simulink model "nms_3Dmodel_inv_wAnkleCPG"  (R2016b)
settings: Solver=ode3  StartTime=0.0  StopTime=tend  FixedStep=ts  RelTol=1e-3  EnableMultiTasking=on
InitFcn:
  | runScripts_inv;
values from neighbouring files (symbols this model uses):
  c = 0.05    [IID_nms_MechInit.m]    (also in nms_MechInit.m)
  c_jointstop = 0.3 / (pi/180)    (= 17.1887338539)    [IID_nms_MechInit.m]    (also in nms_MechInit.m)
  CPG_On = 1    [setCPGPar.m]    (also in setCPGPar_inv.m)
  CtrlPar_FP = [alpha0 alpha_cd alpha_cv]    [setCtrlPar.m]
  CtrlPar_FP_R = [R_hipR0 R_hipR_cd R_hipR_cv]    [setCtrlPar.m]
  CtrlPar_LL = l_clr    [setCtrlPar.m]
  CtrlPar_St = [StPreStim St_M1 St_M2 St_M3 St_M4 St_M5 St_M11]    [setCtrlPar.m]
  CtrlPar_St_R = [R_StPreStim R_St_M1 R_St_M3 R_St_M4]    [setCtrlPar.m]
  CtrlPar_Sw = [SwPreStim SwPhasePari SwPhaseParii SwCtrlPar_H SwCtrlPar_A      SwCtrlPar_Ki SwCtrlPar_Kii SwCtrlPar_Kiii SwCtrlPar_StP]    [setCtrlPar.m]
  CtrlPar_Sw_R = [R_SwPreStim R_Sw_M6]    [setCtrlPar.m]
  CtrlPar_theta0 = parBlCtrl(1)      *1*pi/180    [setCtrlPar.m]
  CtrlPar_Tr = [Tr_St_sup Tr_Sw]    [setCtrlPar.m]
  CtrlPar_Tr_R = [R_Tr_St_sup R_Tr_Sw]    [setCtrlPar.m]
  eref = 0.04    [IID_nms_MechInit.m]    (also in nms_MechInit.m)
  FmaxBFSH = 350    [nms_MechInit.m]
  FmaxGAS = 1500    [IID_nms_MechInit.m]    (also in nms_MechInit.m)
  FmaxGLU = 1500    [IID_nms_MechInit.m]    (also in nms_MechInit.m)
  FmaxHAB = 3000    [nms_MechInit.m]
  FmaxHAD = 4500    [nms_MechInit.m]
  FmaxHAM = 3000    [IID_nms_MechInit.m]    (also in nms_MechInit.m)
  FmaxHFL = 2000    [IID_nms_MechInit.m]    (also in nms_MechInit.m)
  FmaxRF = 1200    [nms_MechInit.m]
  FmaxSOL = 4000    [IID_nms_MechInit.m]    (also in nms_MechInit.m)
  FmaxTA = 800    [IID_nms_MechInit.m]    (also in nms_MechInit.m)
  FmaxVAS = 6000    [IID_nms_MechInit.m]    (also in nms_MechInit.m)
  init_a_tgt = 70*pi/180    (= 1.2217304764)    [setInitPar.m]
  init_a_tgtR = 90*pi/180    (= 1.57079632679)    [setInitPar.m]
  K = 5    [IID_nms_MechInit.m]    (also in nms_MechInit.m)
  leg_l = [D12_T D12_S]    [nms_MechInit.m]
  LongDelay = 0.020    (= 0.02)    [IID_setCtrlPar.m]    (also in nms_MechInit.m = 0.01)
  LongLoopDelay = 0.030    (= 0.03)    [nms_MechInit.m]
  loptBFSH = 0.12    [nms_MechInit.m]
  loptGAS = 0.05    [IID_nms_MechInit.m]    (also in nms_MechInit.m)
  loptGLU = 0.11    [IID_nms_MechInit.m]    (also in nms_MechInit.m)
  loptHAB = 0.09    [nms_MechInit.m]
  loptHAD = 0.10    (= 0.1)    [nms_MechInit.m]
  loptHAM = 0.10    (= 0.1)    [IID_nms_MechInit.m]    (also in nms_MechInit.m)
  loptHFL = 0.11    [IID_nms_MechInit.m]    (also in nms_MechInit.m)
  loptRF = 0.08    [nms_MechInit.m]
  loptSOL = 0.04    [IID_nms_MechInit.m]    (also in nms_MechInit.m)
  loptTA = 0.06    [IID_nms_MechInit.m]    (also in nms_MechInit.m)
  loptVAS = 0.08    [IID_nms_MechInit.m]    (also in nms_MechInit.m)
  lslackBFSH = 0.10    (= 0.1)    [nms_MechInit.m]
  lslackGAS = 0.40    (= 0.4)    [IID_nms_MechInit.m]    (also in nms_MechInit.m)
  lslackGLU = 0.13    [IID_nms_MechInit.m]    (also in nms_MechInit.m)
  lslackHAB = 0.07    [nms_MechInit.m]
  lslackHAD = 0.18    [nms_MechInit.m]
  lslackHAM = 0.31    [IID_nms_MechInit.m]    (also in nms_MechInit.m)
  lslackHFL = 0.10    (= 0.1)    [IID_nms_MechInit.m]    (also in nms_MechInit.m)
  lslackRF = 0.35    [nms_MechInit.m]
  lslackSOL = 0.26    [IID_nms_MechInit.m]    (also in nms_MechInit.m)
  lslackTA = 0.24    [IID_nms_MechInit.m]    (also in nms_MechInit.m)
  lslackVAS = 0.23    [IID_nms_MechInit.m]    (also in nms_MechInit.m)
  massBFSH = 2    [nms_MechInit.m]
  massGAS = 0.45    [IID_nms_MechInit.m]    (also in nms_MechInit.m)
  massGLU = 1.4    [IID_nms_MechInit.m]    (also in nms_MechInit.m)
  massHAB = 1.145    [nms_MechInit.m]
  massHAD = 1.91    [nms_MechInit.m]
  massHAM = 1.82    [IID_nms_MechInit.m]    (also in nms_MechInit.m)
  massHFL = 1.87    [IID_nms_MechInit.m]    (also in nms_MechInit.m)
  massRF = 1    [nms_MechInit.m]
  massSOL = 1.36    [IID_nms_MechInit.m]    (also in nms_MechInit.m)
  massTA = 0.29    [IID_nms_MechInit.m]    (also in nms_MechInit.m)
  massVAS = 2.91    [IID_nms_MechInit.m]    (also in nms_MechInit.m)
  MidDelay = 0.010    (= 0.01)    [IID_setCtrlPar.m]    (also in nms_MechInit.m = 0.005)
  N = 1.5    [IID_nms_MechInit.m]    (also in cmaes_parfor.m = size(x,1); nms_MechInit.m)
  phi12_LowLimit = 70*pi/180    (= 1.2217304764)    [IID_nms_MechInit.m]    (also in nms_MechInit.m)
  phi12_UpLimit = 130*pi/180    (= 2.26892802759)    [IID_nms_MechInit.m]    (also in nms_MechInit.m)
  phi23_UpLimit = 175*pi/180    (= 3.05432619099)    [IID_nms_MechInit.m]    (also in nms_MechInit.m)
  phi34_UpLimit = 230*pi/180    (= 4.01425727959)    [IID_nms_MechInit.m]    (also in nms_MechInit.m)
  phi34R_LowLimit = -15*pi/180    (= -0.261799387799)    [nms_MechInit.m]
  phi34R_UpLimit = 50*pi/180    (= 0.872664625997)    [nms_MechInit.m]
  phimaxGASa = 110*pi/180    (= 1.91986217719)    [IID_nms_MechInit.m]    (also in nms_MechInit.m = 1.74532925199)
  phimaxGASk = 140*pi/180    (= 2.44346095279)    [IID_nms_MechInit.m]    (also in nms_MechInit.m)
  phimaxRFk = 165*pi/180    (= 2.87979326579)    [nms_MechInit.m]
  phimaxSOL = 110*pi/180    (= 1.91986217719)    [IID_nms_MechInit.m]    (also in nms_MechInit.m = 1.74532925199)
  phimaxTA = 80*pi/180    (= 1.3962634016)    [IID_nms_MechInit.m]    (also in nms_MechInit.m)
  phimaxVAS = 165*pi/180    (= 2.87979326579)    [IID_nms_MechInit.m]    (also in nms_MechInit.m)
  phirefBFSH = 160*pi/180    (= 2.79252680319)    [nms_MechInit.m]
  phirefGASa = 80*pi/180    (= 1.3962634016)    [IID_nms_MechInit.m]    (also in nms_MechInit.m)
  phirefGASk = 165*pi/180    (= 2.87979326579)    [IID_nms_MechInit.m]    (also in nms_MechInit.m)
  phirefGLU = 150*pi/180    (= 2.61799387799)    [IID_nms_MechInit.m]    (also in nms_MechInit.m = 2.09439510239)
  phirefHAB = 10*pi/180    (= 0.174532925199)    [nms_MechInit.m]
  phirefHAD = 15*pi/180    (= 0.261799387799)    [nms_MechInit.m]
  phirefHAMh = 155*pi/180    (= 2.70526034059)    [IID_nms_MechInit.m]    (also in nms_MechInit.m = 2.61799387799)
  phirefHAMk = 180*pi/180    (= 3.14159265359)    [IID_nms_MechInit.m]    (also in nms_MechInit.m)
  phirefHFL = 180*pi/180    (= 3.14159265359)    [IID_nms_MechInit.m]    (also in nms_MechInit.m = 2.79252680319)
  phirefRFh = 170*pi/180    (= 2.96705972839)    [nms_MechInit.m]
  phirefRFk = 125*pi/180    (= 2.18166156499)    [nms_MechInit.m]
  phirefSOL = 80*pi/180    (= 1.3962634016)    [IID_nms_MechInit.m]    (also in nms_MechInit.m = 1.57079632679)
  phirefTA = 110*pi/180    (= 1.91986217719)    [IID_nms_MechInit.m]    (also in nms_MechInit.m)
  phirefVAS = 125*pi/180    (= 2.18166156499)    [IID_nms_MechInit.m]    (also in nms_MechInit.m = 2.09439510239)
  phiScaleGASa = acos(rGASamin/rGASamax)/(phiminGASa-phimaxGASa)    [nms_MechInit.m]
  phiScaleGASk = acos(rGASkmin/rGASkmax)/(phiminGASk-phimaxGASk)    [nms_MechInit.m]
  phiScaleRFk = acos(rRFkmin/rRFkmax)/(phiminRFk-phimaxRFk)    [nms_MechInit.m]
  phiScaleSOL = acos(rSOLmin/rSOLmax)/(phiminSOL-phimaxSOL)    [nms_MechInit.m]
  phiScaleTA = acos(rTAmin/rTAmax)/(phiminTA-phimaxTA)    [nms_MechInit.m]
  phiScaleVAS = acos(rVASmin/rVASmax)/(phiminVAS-phimaxVAS)    [nms_MechInit.m]
  rBFSH = 0.04    [nms_MechInit.m]
  rGASamax = 0.06    [nms_MechInit.m]
  rGASkmax = 0.05    [nms_MechInit.m]
  rGLU = 0.10    (= 0.1)    [IID_nms_MechInit.m]    (also in nms_MechInit.m = 0.08)
  rHAB = 0.06    [nms_MechInit.m]
  rHAD = 0.03    [nms_MechInit.m]
  rHAMh = 0.08    [IID_nms_MechInit.m]    (also in nms_MechInit.m)
  rHAMk = 0.05    [IID_nms_MechInit.m]    (also in nms_MechInit.m)
  rHFL = 0.10    (= 0.1)    [IID_nms_MechInit.m]    (also in nms_MechInit.m = 0.08)
  rhoBFSH = 0.7    [nms_MechInit.m]
  rhoGASa = 0.7    [IID_nms_MechInit.m]    (also in nms_MechInit.m)
  rhoGASk = 0.7    [IID_nms_MechInit.m]    (also in nms_MechInit.m)
  rhoGLU = 0.5    [IID_nms_MechInit.m]    (also in nms_MechInit.m)
  rhoHAB = 0.7    [nms_MechInit.m]
  rhoHAD = 1    [nms_MechInit.m]
  rhoHAMh = 0.7    [IID_nms_MechInit.m]    (also in nms_MechInit.m = 0.5)
  rhoHAMk = 0.7    [IID_nms_MechInit.m]    (also in nms_MechInit.m = 0.5)
  rhoHFL = 0.5    [IID_nms_MechInit.m]    (also in nms_MechInit.m)
  rhoRFh = 0.3    [nms_MechInit.m]
  rhoRFk = 0.5    [nms_MechInit.m]
  rhoSOL = 0.5    [IID_nms_MechInit.m]    (also in nms_MechInit.m)
  rhoTA = 0.7    [IID_nms_MechInit.m]    (also in nms_MechInit.m)
  ... (+55 more)
libraries: simulink_extras x30, nmc x30, simulink x22, NMCCPG_Library x13, powerlib_meascontrol x5
(part 4 of 12)

== system nms_3Dmodel_inv_wAnkleCPG/NMC Model/Muscle Actuation Layer/L GLU ==
  note: Excitation Contraction Coupling
  note: GLU Muscle-Tendon Dynamics
  STIM : Inport
  lmtc [m] : Inport  Port=2
  1 : Product  Inputs=**  SaturateOnIntegerOverflow=on  InputSameDT=on  OutDataTypeStr=Inherit: Same as first input
  1/lslack : Gain  Gain=1/lslackGLU  SaturateOnIntegerOverflow=on  OutDataTypeStr=Inherit: Same as input  ParamDataTypeStr=Inherit: Same as input
  2 : Product  Inputs=***  SaturateOnIntegerOverflow=on  InputSameDT=on  OutDataTypeStr=Inherit: Same as first input
  BE force-length relation : Subsystem
  CE force-length relation : Subsystem
  CE inverse force-velocity relation : Subsystem
  Constant : Constant  Value=lslackGLU
  ECC TransferFcn : simulink_extras/Additional Linear/Transfer Fcn (with initial outputs)  N=[1]  D="[tau  1]"  Y0=preA  U0=0
      settings: AttributesFormatString=pre-activation: %<Y0>
  Fmax : Gain  Gain=FmaxGLU  SaturateOnIntegerOverflow=on  OutDataTypeStr=Inherit: Same as input  ParamDataTypeStr=Inherit: Same as input
  Fmax1 : Gain  Gain=FmaxGLU  SaturateOnIntegerOverflow=on  OutDataTypeStr=Inherit: Same as input  ParamDataTypeStr=Inherit: Same as input
  Fv = Fse / (A*Fce) : Product  Inputs=*/  SaturateOnIntegerOverflow=on  InputSameDT=on  OutDataTypeStr=Inherit: Same as first input
  Integrator : Integrator  InitialConditionSource=external  LowerSaturationLimit=0.05  ZeroCross=off
  PE force-length relation : Subsystem
  SE force-length relation : Subsystem
  Sum : Sum  Inputs=|+-  SaturateOnIntegerOverflow=on  InputSameDT=on  OutDataTypeStr=Inherit: Same as first input
  Sum2 : Sum  Inputs=|-+  SaturateOnIntegerOverflow=on  InputSameDT=on  OutDataTypeStr=Inherit: Same as first input
  Sum3 : Sum  SaturateOnIntegerOverflow=on  InputSameDT=on  OutDataTypeStr=Inherit: Same as first input
  Sum4 : Sum  SaturateOnIntegerOverflow=on  InputSameDT=on  OutDataTypeStr=Inherit: Same as first input
  lce/lopt : Gain  Gain=1/loptGLU  SaturateOnIntegerOverflow=on  OutDataTypeStr=Inherit: Same as input  ParamDataTypeStr=Inherit: Same as input
  vmax*lopt : Gain  Gain=vmaxGLU*loptGLU  SaturateOnIntegerOverflow=on  OutDataTypeStr=Inherit: Same as input  ParamDataTypeStr=Inherit: Same as input
  Fmtc : Outport  InitialOutput=0
  Lce : Outport  Port=2  InitialOutput=0
  Vce : Outport  Port=3  InitialOutput=0
  A : Outport  Port=4  InitialOutput=0
  Fac : Outport  Port=5  InitialOutput=0
  wires:
  Fmax1/1 -> Fac/1
  2/1 -> Fmax1/1
  ECC TransferFcn/1 -> 1/2, A/1, 2/2  "A"
  CE force-length relation/1(fce [Fmax]) -> 1/1, 2/1  "fl"
  Fv = Fse / (A*Fce)/1 -> CE inverse force-velocity relation/1(Fv[Fmax]), 2/3  "fv"
  STIM/1 -> ECC TransferFcn/1
  CE inverse force-velocity relation/1(v[vmax]) -> vmax*lopt/1
  Sum3/1 -> Fv = Fse / (A*Fce)/2
  BE force-length relation/1(fbe [Fmax]) -> Sum4/2
  1/1 -> Sum3/2
  PE force-length relation/1(fpe [Fmax]) -> Sum3/1
  Sum4/1 -> Fv = Fse / (A*Fce)/1
  Constant/1 -> Sum2/1
  Sum2/1 -> Integrator/2
  SE force-length relation/1(fse [Fmax]) -> Sum4/1, Fmax/1
  1/lslack/1 -> SE force-length relation/1(lse [lslack])
  Fmax/1 -> Fmtc/1  "Fmtc"
  lmtc [m]/1 -> Sum/1, Sum2/2  "lmtc"
  vmax*lopt/1 -> Vce/1, Integrator/1  "vce"
  lce/lopt/1 -> PE force-length relation/1(lce [lopt]), BE force-length relation/1(lce [lopt]), CE force-length relation/1(lce [lopt])
  Sum/1 -> 1/lslack/1  "lse"
  Integrator/1 -> Lce/1, lce/lopt/1, Sum/2  "lce"

== system nms_3Dmodel_inv_wAnkleCPG/NMC Model/Muscle Actuation Layer/L GLU Link ==
  note: GLUTEUS Attachment
  phi34 [rad] : Inport
  Constant : Constant  Value=lslackGLU+loptGLU
  Constant1 : Constant  Value=rGLU
  Constant2 : Constant  Value=phirefGLU
  Gain2 : Gain  Gain=rhoGLU
  Product : Product  RndMeth=Zero
  Sum2 : Sum  Inputs=|+-
  Sum5 : Sum  Inputs=|+-
  lmtu [m] : Outport
  lever [m] : Outport  Port=2
  wires:
  Gain2/1 -> Sum5/2
  Constant1/1 -> lever [m]/1, Product/2
  Sum2/1 -> Product/1
  Constant2/1 -> Sum2/2
  phi34 [rad]/1 -> Sum2/1
  Product/1 -> Gain2/1
  Sum5/1 -> lmtu [m]/1
  Constant/1 -> Sum5/1

== system nms_3Dmodel_inv_wAnkleCPG/NMC Model/Muscle Actuation Layer/L HAB ==
  note: HAB Muscle-Tendon Dynamics
  note: Excitation Contraction Coupling
  STIM : Inport
  lmtc [m] : Inport  Port=2
  1 : Product  Inputs=**  SaturateOnIntegerOverflow=on  InputSameDT=on  OutDataTypeStr=Inherit: Same as first input
  1/lslack : Gain  Gain=1/lslackHAB  SaturateOnIntegerOverflow=on  OutDataTypeStr=Inherit: Same as input  ParamDataTypeStr=Inherit: Same as input
  2 : Product  Inputs=***  SaturateOnIntegerOverflow=on  InputSameDT=on  OutDataTypeStr=Inherit: Same as first input
  BE force-length relation : Subsystem
  CE force-length relation : Subsystem
  CE inverse force-velocity relation : Subsystem
  Constant : Constant  Value=lslackHAB
  ECC TransferFcn : simulink_extras/Additional Linear/Transfer Fcn (with initial outputs)  N=[1]  D="[tau  1]"  Y0=preA  U0=0
      settings: AttributesFormatString=pre-activation: %<Y0>
  Fmax : Gain  Gain=FmaxHAB  SaturateOnIntegerOverflow=on  OutDataTypeStr=Inherit: Same as input  ParamDataTypeStr=Inherit: Same as input
  Fmax1 : Gain  Gain=FmaxHAB  SaturateOnIntegerOverflow=on  OutDataTypeStr=Inherit: Same as input  ParamDataTypeStr=Inherit: Same as input
  Fv = Fse / (A*Fce) : Product  Inputs=*/  SaturateOnIntegerOverflow=on  InputSameDT=on  OutDataTypeStr=Inherit: Same as first input
  Integrator : Integrator  InitialConditionSource=external  LowerSaturationLimit=0.05  ZeroCross=off
  PE force-length relation : Subsystem
  SE force-length relation : Subsystem
  Sum : Sum  Inputs=|+-  SaturateOnIntegerOverflow=on  InputSameDT=on  OutDataTypeStr=Inherit: Same as first input
  Sum2 : Sum  Inputs=|-+  SaturateOnIntegerOverflow=on  InputSameDT=on  OutDataTypeStr=Inherit: Same as first input
  Sum3 : Sum  SaturateOnIntegerOverflow=on  InputSameDT=on  OutDataTypeStr=Inherit: Same as first input
  Sum4 : Sum  SaturateOnIntegerOverflow=on  InputSameDT=on  OutDataTypeStr=Inherit: Same as first input
  lce/lopt : Gain  Gain=1/loptHAB  SaturateOnIntegerOverflow=on  OutDataTypeStr=Inherit: Same as input  ParamDataTypeStr=Inherit: Same as input
  vmax*lopt : Gain  Gain=vmaxHAB*loptHAB  SaturateOnIntegerOverflow=on  OutDataTypeStr=Inherit: Same as input  ParamDataTypeStr=Inherit: Same as input
  Fmtc : Outport  InitialOutput=0
  Lce : Outport  Port=2  InitialOutput=0
  Vce : Outport  Port=3  InitialOutput=0
  A : Outport  Port=4  InitialOutput=0
  Fac : Outport  Port=5  InitialOutput=0
  wires:
  Integrator/1 -> Sum/2, lce/lopt/1, Lce/1  "lce"
  Sum/1 -> 1/lslack/1  "lse"
  lce/lopt/1 -> CE force-length relation/1(lce [lopt]), BE force-length relation/1(lce [lopt]), PE force-length relation/1(lce [lopt])
  vmax*lopt/1 -> Integrator/1, Vce/1  "vce"
  lmtc [m]/1 -> Sum2/2, Sum/1  "lmtc"
  Fmax/1 -> Fmtc/1  "Fmtc"
  1/lslack/1 -> SE force-length relation/1(lse [lslack])
  SE force-length relation/1(fse [Fmax]) -> Fmax/1, Sum4/1
  Sum2/1 -> Integrator/2
  Constant/1 -> Sum2/1
  Sum4/1 -> Fv = Fse / (A*Fce)/1
  PE force-length relation/1(fpe [Fmax]) -> Sum3/1
  1/1 -> Sum3/2
  BE force-length relation/1(fbe [Fmax]) -> Sum4/2
  Sum3/1 -> Fv = Fse / (A*Fce)/2
  CE inverse force-velocity relation/1(v[vmax]) -> vmax*lopt/1
  STIM/1 -> ECC TransferFcn/1
  Fv = Fse / (A*Fce)/1 -> 2/3, CE inverse force-velocity relation/1(Fv[Fmax])  "fv"
  CE force-length relation/1(fce [Fmax]) -> 2/1, 1/1  "fl"
  ECC TransferFcn/1 -> 2/2, A/1, 1/2  "A"
  2/1 -> Fmax1/1
  Fmax1/1 -> Fac/1

== system nms_3Dmodel_inv_wAnkleCPG/NMC Model/Muscle Actuation Layer/L HAB Link ==
  note: HAB Attachment
  phi34R [rad] : Inport
  Constant : Constant  Value=lslackHAB+loptHAB
  Constant1 : Constant  Value=rHAB
  Constant2 : Constant  Value=phirefHAB
  Gain2 : Gain  Gain=rhoHAB
  Product : Product  RndMeth=Zero
  Sum2 : Sum  Inputs=|+-
  Sum5 : Sum  Inputs=|+-
  lmtu [m] : Outport
  lever [m] : Outport  Port=2
  wires:
  Gain2/1 -> Sum5/2
  Constant1/1 -> lever [m]/1, Product/2
  Sum2/1 -> Product/1
  Constant2/1 -> Sum2/2
  phi34R [rad]/1 -> Sum2/1
  Product/1 -> Gain2/1
  Sum5/1 -> lmtu [m]/1
  Constant/1 -> Sum5/1

== system nms_3Dmodel_inv_wAnkleCPG/NMC Model/Muscle Actuation Layer/L HAD ==
  note: HAD Muscle-Tendon Dynamics
  note: Excitation Contraction Coupling
  STIM : Inport
  lmtc [m] : Inport  Port=2
  1 : Product  Inputs=**  SaturateOnIntegerOverflow=on  InputSameDT=on  OutDataTypeStr=Inherit: Same as first input
  1/lslack : Gain  Gain=1/lslackHAD  SaturateOnIntegerOverflow=on  OutDataTypeStr=Inherit: Same as input  ParamDataTypeStr=Inherit: Same as input
  2 : Product  Inputs=***  SaturateOnIntegerOverflow=on  InputSameDT=on  OutDataTypeStr=Inherit: Same as first input
  BE force-length relation : Subsystem
  CE force-length relation : Subsystem
  CE inverse force-velocity relation : Subsystem
  Constant : Constant  Value=lslackHAD
  ECC TransferFcn : simulink_extras/Additional Linear/Transfer Fcn (with initial outputs)  N=[1]  D="[tau  1]"  Y0=preA  U0=0
      settings: AttributesFormatString=pre-activation: %<Y0>
  Fmax : Gain  Gain=FmaxHAD  SaturateOnIntegerOverflow=on  OutDataTypeStr=Inherit: Same as input  ParamDataTypeStr=Inherit: Same as input
  Fmax1 : Gain  Gain=FmaxHAD  SaturateOnIntegerOverflow=on  OutDataTypeStr=Inherit: Same as input  ParamDataTypeStr=Inherit: Same as input
  Fv = Fse / (A*Fce) : Product  Inputs=*/  SaturateOnIntegerOverflow=on  InputSameDT=on  OutDataTypeStr=Inherit: Same as first input
  Integrator : Integrator  InitialConditionSource=external  LowerSaturationLimit=0.05  ZeroCross=off
  PE force-length relation : Subsystem
  SE force-length relation : Subsystem
  Sum : Sum  Inputs=|+-  SaturateOnIntegerOverflow=on  InputSameDT=on  OutDataTypeStr=Inherit: Same as first input
  Sum2 : Sum  Inputs=|-+  SaturateOnIntegerOverflow=on  InputSameDT=on  OutDataTypeStr=Inherit: Same as first input
  Sum3 : Sum  SaturateOnIntegerOverflow=on  InputSameDT=on  OutDataTypeStr=Inherit: Same as first input
  Sum4 : Sum  SaturateOnIntegerOverflow=on  InputSameDT=on  OutDataTypeStr=Inherit: Same as first input
  lce/lopt : Gain  Gain=1/loptHAD  SaturateOnIntegerOverflow=on  OutDataTypeStr=Inherit: Same as input  ParamDataTypeStr=Inherit: Same as input
  vmax*lopt : Gain  Gain=vmaxHAD*loptHAD  SaturateOnIntegerOverflow=on  OutDataTypeStr=Inherit: Same as input  ParamDataTypeStr=Inherit: Same as input
  Fmtc : Outport  InitialOutput=0
  Lce : Outport  Port=2  InitialOutput=0
  Vce : Outport  Port=3  InitialOutput=0
  A : Outport  Port=4  InitialOutput=0
  Fac : Outport  Port=5  InitialOutput=0
  wires:
  Integrator/1 -> Sum/2, lce/lopt/1, Lce/1  "lce"
  Sum/1 -> 1/lslack/1  "lse"
  lce/lopt/1 -> CE force-length relation/1(lce [lopt]), BE force-length relation/1(lce [lopt]), PE force-length relation/1(lce [lopt])
  vmax*lopt/1 -> Integrator/1, Vce/1  "vce"
  lmtc [m]/1 -> Sum2/2, Sum/1  "lmtc"
  Fmax/1 -> Fmtc/1  "Fmtc"
  1/lslack/1 -> SE force-length relation/1(lse [lslack])
  SE force-length relation/1(fse [Fmax]) -> Fmax/1, Sum4/1
  Sum2/1 -> Integrator/2
  Constant/1 -> Sum2/1
  CE force-length relation/1(fce [Fmax]) -> 2/1, 1/1
  Sum4/1 -> Fv = Fse / (A*Fce)/1
  PE force-length relation/1(fpe [Fmax]) -> Sum3/1
  1/1 -> Sum3/2
  BE force-length relation/1(fbe [Fmax]) -> Sum4/2
  Sum3/1 -> Fv = Fse / (A*Fce)/2
  CE inverse force-velocity relation/1(v[vmax]) -> vmax*lopt/1
  STIM/1 -> ECC TransferFcn/1
  Fv = Fse / (A*Fce)/1 -> 2/3, CE inverse force-velocity relation/1(Fv[Fmax])  "fv"
  ECC TransferFcn/1 -> 2/2, A/1, 1/2  "A"
  2/1 -> Fmax1/1
  Fmax1/1 -> Fac/1

== system nms_3Dmodel_inv_wAnkleCPG/NMC Model/Muscle Actuation Layer/L HAD Link ==
  note: HAD Attachment
  phi34R [rad] : Inport
  Constant : Constant  Value=lslackHAD+loptHAD
  Constant1 : Constant  Value=rHAD
  Constant2 : Constant  Value=phirefHAD
  Gain2 : Gain  Gain=rhoHAD
  Product : Product  RndMeth=Zero
  Sum2 : Sum  Inputs=|+-
  Sum5 : Sum  Inputs=|++
  lmtu [m] : Outport
  lever [m] : Outport  Port=2
  wires:
  Gain2/1 -> Sum5/2
  Constant1/1 -> lever [m]/1, Product/2
  Sum2/1 -> Product/1
  Constant2/1 -> Sum2/2
  phi34R [rad]/1 -> Sum2/1
  Product/1 -> Gain2/1
  Sum5/1 -> lmtu [m]/1
  Constant/1 -> Sum5/1

== system nms_3Dmodel_inv_wAnkleCPG/NMC Model/Muscle Actuation Layer/L HAM ==
  note: Excitation Contraction Coupling
  note: HAM Muscle-Tendon Dynamics
  STIM : Inport
  lmtc [m] : Inport  Port=2
  1 : Product  Inputs=**  SaturateOnIntegerOverflow=on  InputSameDT=on  OutDataTypeStr=Inherit: Same as first input
  1/lslack : Gain  Gain=1/lslackHAM  SaturateOnIntegerOverflow=on  OutDataTypeStr=Inherit: Same as input  ParamDataTypeStr=Inherit: Same as input
  2 : Product  Inputs=***  SaturateOnIntegerOverflow=on  InputSameDT=on  OutDataTypeStr=Inherit: Same as first input
  BE force-length relation : Subsystem
  CE force-length relation : Subsystem
  CE inverse force-velocity relation : Subsystem
  Constant : Constant  Value=lslackHAM
  ECC TransferFcn : simulink_extras/Additional Linear/Transfer Fcn (with initial outputs)  N=[1]  D="[tau  1]"  Y0=preA  U0=0
      settings: AttributesFormatString=pre-activation: %<Y0>
  Fmax : Gain  Gain=FmaxHAM  SaturateOnIntegerOverflow=on  OutDataTypeStr=Inherit: Same as input  ParamDataTypeStr=Inherit: Same as input
  Fmax1 : Gain  Gain=FmaxHAM  SaturateOnIntegerOverflow=on  OutDataTypeStr=Inherit: Same as input  ParamDataTypeStr=Inherit: Same as input
  Fv = Fse / (A*Fce) : Product  Inputs=*/  SaturateOnIntegerOverflow=on  InputSameDT=on  OutDataTypeStr=Inherit: Same as first input
  Integrator : Integrator  InitialConditionSource=external  LowerSaturationLimit=0.05  ZeroCross=off
  PE force-length relation : Subsystem
  SE force-length relation : Subsystem
  Sum : Sum  Inputs=|+-  SaturateOnIntegerOverflow=on  InputSameDT=on  OutDataTypeStr=Inherit: Same as first input
  Sum2 : Sum  Inputs=|-+  SaturateOnIntegerOverflow=on  InputSameDT=on  OutDataTypeStr=Inherit: Same as first input
  Sum3 : Sum  SaturateOnIntegerOverflow=on  InputSameDT=on  OutDataTypeStr=Inherit: Same as first input
  Sum4 : Sum  SaturateOnIntegerOverflow=on  InputSameDT=on  OutDataTypeStr=Inherit: Same as first input
  lce/lopt : Gain  Gain=1/loptHAM  SaturateOnIntegerOverflow=on  OutDataTypeStr=Inherit: Same as input  ParamDataTypeStr=Inherit: Same as input
  vmax*lopt : Gain  Gain=vmaxHAM*loptHAM  SaturateOnIntegerOverflow=on  OutDataTypeStr=Inherit: Same as input  ParamDataTypeStr=Inherit: Same as input
  Fmtc : Outport  InitialOutput=0
  Lce : Outport  Port=2  InitialOutput=0
  Vce : Outport  Port=3  InitialOutput=0
  A : Outport  Port=4  InitialOutput=0
  Fac : Outport  Port=5  InitialOutput=0
  wires:
  Fmax1/1 -> Fac/1
  2/1 -> Fmax1/1
  ECC TransferFcn/1 -> A/1, 2/2, 1/2  "A"
  CE force-length relation/1(fce [Fmax]) -> 1/1, 2/1  "fl"
  Fv = Fse / (A*Fce)/1 -> CE inverse force-velocity relation/1(Fv[Fmax]), 2/3  "fv"
  STIM/1 -> ECC TransferFcn/1
  CE inverse force-velocity relation/1(v[vmax]) -> vmax*lopt/1
  Sum3/1 -> Fv = Fse / (A*Fce)/2
  BE force-length relation/1(fbe [Fmax]) -> Sum4/2
  1/1 -> Sum3/2
  PE force-length relation/1(fpe [Fmax]) -> Sum3/1
  Sum4/1 -> Fv = Fse / (A*Fce)/1
  Constant/1 -> Sum2/1
  Sum2/1 -> Integrator/2
  SE force-length relation/1(fse [Fmax]) -> Sum4/1, Fmax/1
  1/lslack/1 -> SE force-length relation/1(lse [lslack])
  Fmax/1 -> Fmtc/1  "Fmtc"
  lmtc [m]/1 -> Sum/1, Sum2/2  "lmtc"
  vmax*lopt/1 -> Vce/1, Integrator/1  "vce"
  lce/lopt/1 -> PE force-length relation/1(lce [lopt]), BE force-length relation/1(lce [lopt]), CE force-length relation/1(lce [lopt])
  Sum/1 -> 1/lslack/1  "lse"
  Integrator/1 -> Lce/1, lce/lopt/1, Sum/2  "lce"

== system nms_3Dmodel_inv_wAnkleCPG/NMC Model/Muscle Actuation Layer/L HAM Link ==
  note: HAM Attachment
  phi34 [rad] : Inport
  phi23 [rad] : Inport  Port=2
  Constant1 : Constant  Value=rHAMk
  Constant2 : Constant  Value=phirefHAMk
  Constant3 : Constant  Value=rHAMh
  Constant4 : Constant  Value=lslackHAM+loptHAM
  Constant5 : Constant  Value=phirefHAMh
  Gain2 : Gain  Gain=rhoHAMh
  Gain4 : Gain  Gain=rhoHAMk
  Product : Product  RndMeth=Zero
  Product1 : Product  RndMeth=Zero
  Sum1 : Sum  Inputs=|+-
  Sum4 : Sum  Inputs=|+-
  Sum5 : Sum  Inputs=-++
  lmtu [m] : Outport
  lever34 [m] : Outport  Port=2
  lever23 [m] : Outport  Port=3
  wires:
  Product1/1 -> Gain4/1
  Constant1/1 -> lever23 [m]/1, Product1/2
  Sum1/1 -> Product1/1
  Constant2/1 -> Sum1/2
  phi23 [rad]/1 -> Sum1/1
  Product/1 -> Gain2/1
  Constant3/1 -> lever34 [m]/1, Product/2
  Sum4/1 -> Product/1
  Constant5/1 -> Sum4/2
  phi34 [rad]/1 -> Sum4/1
  Gain2/1 -> Sum5/1
  Gain4/1 -> Sum5/3
  Constant4/1 -> Sum5/2
  Sum5/1 -> lmtu [m]/1

== system nms_3Dmodel_inv_wAnkleCPG/NMC Model/Muscle Actuation Layer/L HFL ==
  note: Excitation Contraction Coupling
  note: HFL Muscle-Tendon Dynamics
  STIM : Inport
  lmtc [m] : Inport  Port=2
  1 : Product  Inputs=**  SaturateOnIntegerOverflow=on  InputSameDT=on  OutDataTypeStr=Inherit: Same as first input
  1/lslack : Gain  Gain=1/lslackHFL  SaturateOnIntegerOverflow=on  OutDataTypeStr=Inherit: Same as input  ParamDataTypeStr=Inherit: Same as input
  2 : Product  Inputs=***  SaturateOnIntegerOverflow=on  InputSameDT=on  OutDataTypeStr=Inherit: Same as first input
  BE force-length relation : Subsystem
  CE force-length relation : Subsystem
  CE inverse force-velocity relation : Subsystem
  Constant : Constant  Value=lslackHFL
  ECC TransferFcn : simulink_extras/Additional Linear/Transfer Fcn (with initial outputs)  N=[1]  D="[tau  1]"  Y0=preA  U0=0
      settings: AttributesFormatString=pre-activation: %<Y0>
  Fmax : Gain  Gain=FmaxHFL  SaturateOnIntegerOverflow=on  OutDataTypeStr=Inherit: Same as input  ParamDataTypeStr=Inherit: Same as input
  Fmax1 : Gain  Gain=FmaxHFL  SaturateOnIntegerOverflow=on  OutDataTypeStr=Inherit: Same as input  ParamDataTypeStr=Inherit: Same as input
  Fv = Fse / (A*Fce) : Product  Inputs=*/  SaturateOnIntegerOverflow=on  InputSameDT=on  OutDataTypeStr=Inherit: Same as first input
  Integrator : Integrator  InitialConditionSource=external  LowerSaturationLimit=0.05  ZeroCross=off
  PE force-length relation : Subsystem
  SE force-length relation : Subsystem
  Sum : Sum  Inputs=|+-  SaturateOnIntegerOverflow=on  InputSameDT=on  OutDataTypeStr=Inherit: Same as first input
  Sum2 : Sum  Inputs=|-+  SaturateOnIntegerOverflow=on  InputSameDT=on  OutDataTypeStr=Inherit: Same as first input
  Sum3 : Sum  SaturateOnIntegerOverflow=on  InputSameDT=on  OutDataTypeStr=Inherit: Same as first input
  Sum4 : Sum  SaturateOnIntegerOverflow=on  InputSameDT=on  OutDataTypeStr=Inherit: Same as first input
  lce/lopt : Gain  Gain=1/loptHFL  SaturateOnIntegerOverflow=on  OutDataTypeStr=Inherit: Same as input  ParamDataTypeStr=Inherit: Same as input
  vmax*lopt : Gain  Gain=vmaxHFL*loptHFL  SaturateOnIntegerOverflow=on  OutDataTypeStr=Inherit: Same as input  ParamDataTypeStr=Inherit: Same as input
  Fmtc : Outport  InitialOutput=0
  Lce : Outport  Port=2  InitialOutput=0
  Vce : Outport  Port=3  InitialOutput=0
  A : Outport  Port=4  InitialOutput=0
  Fac : Outport  Port=5  InitialOutput=0
  wires:
  Fmax1/1 -> Fac/1
  2/1 -> Fmax1/1
  ECC TransferFcn/1 -> 1/2, A/1, 2/2  "A"
  STIM/1 -> ECC TransferFcn/1
  CE inverse force-velocity relation/1(v[vmax]) -> vmax*lopt/1
  Sum3/1 -> Fv = Fse / (A*Fce)/2
  BE force-length relation/1(fbe [Fmax]) -> Sum4/2  "Fbe"
  1/1 -> Sum3/2
  PE force-length relation/1(fpe [Fmax]) -> Sum3/1  "Fpe"
  Sum4/1 -> Fv = Fse / (A*Fce)/1
  CE force-length relation/1(fce [Fmax]) -> 1/1, 2/1  "fl"
  Constant/1 -> Sum2/1
  Sum2/1 -> Integrator/2
  SE force-length relation/1(fse [Fmax]) -> Fmax/1, Sum4/1  "Fse"
  1/lslack/1 -> SE force-length relation/1(lse [lslack])
  Fmax/1 -> Fmtc/1  "Fmtc"
  lmtc [m]/1 -> Sum/1, Sum2/2  "lmtc"
  vmax*lopt/1 -> Vce/1, Integrator/1  "vce"
  Fv = Fse / (A*Fce)/1 -> CE inverse force-velocity relation/1(Fv[Fmax]), 2/3  "fv"
  lce/lopt/1 -> PE force-length relation/1(lce [lopt]), BE force-length relation/1(lce [lopt]), CE force-length relation/1(lce [lopt])
  Sum/1 -> 1/lslack/1  "lse"
  Integrator/1 -> Lce/1, lce/lopt/1, Sum/2  "lce"

== system nms_3Dmodel_inv_wAnkleCPG/NMC Model/Muscle Actuation Layer/L HFL Link ==
  note: HFL Attachment
  phi34 [rad] : Inport
  Constant : Constant  Value=lslackHFL+loptHFL
  Constant1 : Constant  Value=rHFL
  Constant2 : Constant  Value=phirefHFL
  Gain2 : Gain  Gain=rhoHFL
  Product : Product  RndMeth=Zero
  Sum2 : Sum  Inputs=|+-
  Sum5 : Sum  Inputs=|++
  lmtu [m] : Outport
  lever [m] : Outport  Port=2
  wires:
  Gain2/1 -> Sum5/2
  Constant1/1 -> lever [m]/1, Product/2
  Sum2/1 -> Product/1
  Constant2/1 -> Sum2/2
  phi34 [rad]/1 -> Sum2/1
  Product/1 -> Gain2/1
  Sum5/1 -> lmtu [m]/1
  Constant/1 -> Sum5/1

== system nms_3Dmodel_inv_wAnkleCPG/NMC Model/Muscle Actuation Layer/L Hip Joint Limits ==
  note: Ankle Joint Limits
  phi [rad] : Inport
  dphi [rad/s] : Inport  Port=2
  Gain2 : Gain  Gain=-1
  Gain3 : Gain  Gain=c_jointstop
  Gain4 : Gain  Gain=1/w_max_jointstop
  Limit Ankle Range : simulink/Logic and Bit Operations/Interval Test  IntervalClosedRight=on  uplimit=phi34_UpLimit + 30*pi/180  IntervalClosedLeft=on  lowlimit=10*pi/180  OutDataTypeStr=boolean
  Logical Operator3 : Logic  Operator=NOT  AllPortsSameDT=off  OutDataTypeStr=boolean
  Mux3 : Mux  Inputs=2
  Overextension Torque : Fcn  Expr="- u(1)  *  (1-u(2)) * (u(2)<1) * (u(1)>0)"
  Stop Simulation1 : Stop
  Sum : Sum  Inputs=|+-
  overextension angle : Constant  Value=phi34_UpLimit
  M_stop [Nm] : Outport
  wires:
  Logical Operator3/1 -> Stop Simulation1/1
  Limit Ankle Range/1 -> Logical Operator3/1
  Overextension Torque/1 -> M_stop [Nm]/1
  Gain2/1 -> Mux3/2
  Gain4/1 -> Gain2/1
  Sum/1 -> Gain3/1
  phi [rad]/1 -> Limit Ankle Range/1, Sum/1
  overextension angle/1 -> Sum/2
  dphi [rad/s]/1 -> Gain4/1
  Gain3/1 -> Mux3/1
  Mux3/1 -> Overextension Torque/1

== system nms_3Dmodel_inv_wAnkleCPG/NMC Model/Muscle Actuation Layer/L Hip Roll Joint Limits ==
  note: Ankle Joint Limits
  phi [rad] : Inport
  dphi [rad/s] : Inport  Port=2
  Gain1 : Gain  Gain=c_jointstop
  Gain2 : Gain  Gain=-1
  Gain3 : Gain  Gain=c_jointstop
  Gain4 : Gain  Gain=1/w_max_jointstop
  Limit Ankle Range : simulink/Logic and Bit Operations/Interval Test  IntervalClosedRight=on  uplimit=phi34R_UpLimit + 20*pi/180  IntervalClosedLeft=on  lowlimit=phi34R_LowLimit - 10*pi/180  OutDataTypeStr=boolean
  Logical Operator3 : Logic  Operator=NOT  AllPortsSameDT=off  OutDataTypeStr=boolean
  Mux1 : Mux  Inputs=2
  Mux3 : Mux  Inputs=2
  Overextension Torque : Fcn  Expr="- u(1)  *  (1-u(2)) * (u(2)<1) * (u(1)>0)"
  Overflexion Torque : Fcn  Expr="- u(1)  *  (1-u(2)) * (u(2)<1) * (u(1)<0)"
  Stop Simulation1 : Stop
  Sum : Sum  Inputs=|+-
  Sum1 : Sum  Inputs=|+-
  Sum2 : Sum
  overextension angle : Constant  Value=phi34R_UpLimit
  overflexion angle : Constant  Value=phi34R_LowLimit
  M_stop [Nm] : Outport
  wires:
  Logical Operator3/1 -> Stop Simulation1/1
  Limit Ankle Range/1 -> Logical Operator3/1
  Overextension Torque/1 -> Sum2/1
  Overflexion Torque/1 -> Sum2/2
  Gain2/1 -> Mux3/2
  Sum2/1 -> M_stop [Nm]/1
  Mux1/1 -> Overflexion Torque/1
  overflexion angle/1 -> Sum1/2
  Sum1/1 -> Gain1/1
  Gain1/1 -> Mux1/1
  Gain4/1 -> Mux1/2, Gain2/1
  Sum/1 -> Gain3/1
  phi [rad]/1 -> Limit Ankle Range/1, Sum1/1, Sum/1
  overextension angle/1 -> Sum/2
  dphi [rad/s]/1 -> Gain4/1
  Gain3/1 -> Mux3/1
  Mux3/1 -> Overextension Torque/1

== system nms_3Dmodel_inv_wAnkleCPG/NMC Model/Muscle Actuation Layer/L Knee Joint Limits ==
  note: Ankle Joint Limits
  phi [rad] : Inport
  dphi [rad/s] : Inport  Port=2
  Gain2 : Gain  Gain=-1
  Gain3 : Gain  Gain=c_jointstop
  Gain4 : Gain  Gain=1/w_max_jointstop
  Limit Ankle Range : simulink/Logic and Bit Operations/Interval Test  IntervalClosedRight=on  uplimit=185*pi/180  IntervalClosedLeft=on  lowlimit=40*pi/180  OutDataTypeStr=boolean
  Logical Operator3 : Logic  Operator=NOT  AllPortsSameDT=off  OutDataTypeStr=boolean
  Mux3 : Mux  Inputs=2
  Overextension Torque : Fcn  Expr="- u(1)  *  (1-u(2)) * (u(2)<1) * (u(1)>0)"
  Stop Simulation1 : Stop
  Sum : Sum  Inputs=|+-
  overextension angle : Constant  Value=phi23_UpLimit
  M_stop [Nm] : Outport
  wires:
  Logical Operator3/1 -> Stop Simulation1/1
  Limit Ankle Range/1 -> Logical Operator3/1
  Overextension Torque/1 -> M_stop [Nm]/1
  Gain2/1 -> Mux3/2
  Gain4/1 -> Gain2/1
  Sum/1 -> Gain3/1
  phi [rad]/1 -> Limit Ankle Range/1, Sum/1
  overextension angle/1 -> Sum/2
  dphi [rad/s]/1 -> Gain4/1
  Gain3/1 -> Mux3/1
  Mux3/1 -> Overextension Torque/1

== system nms_3Dmodel_inv_wAnkleCPG/NMC Model/Muscle Actuation Layer/L RF Link ==
  note: RF Attachment
  phi34 [rad] : Inport
  phi23 [rad] : Inport  Port=2
  Constant1 : Constant  Value=phimaxRFk
  Constant2 : Constant  Value=phirefRFk
  Constant3 : Constant  Value=rRFh
  Constant4 : Constant  Value=lslackRF+loptRF
  Constant5 : Constant  Value=phirefRFh
  Demux : Demux  Outputs=2
  Gain1 : Gain  Gain=rRFkmax
  Gain2 : Gain  Gain=rhoRFh
  Gain3 : Gain  Gain=phiScaleRFk
  Gain4 : Gain  Gain=rhoRFk/phiScaleRFk
  Gain5 : Gain  Gain=phiScaleRFk
  Mux : Mux  Inputs=2
  Product : Product  RndMeth=Zero
  Sum1 : Sum  Inputs=-+
  Sum2 : Sum  Inputs=|+-
  Sum3 : Sum  Inputs=-+|
  Sum4 : Sum  Inputs=|+-
  Sum5 : Sum  Inputs=++-
  length change term : Trigonometry
  offset correction term : Trigonometry
  variable lever term : Trigonometry  Operator=cos
  lmtu [m] : Outport
  lever34 [m] : Outport  Port=2
  lever23 [m] : Outport  Port=3
  wires:
  Gain5/1 -> offset correction term/1
  Gain3/1 -> length change term/1, variable lever term/1
  Demux/1 -> Gain4/1
  Demux/2 -> lever23 [m]/1
  Gain1/1 -> Demux/1
  Mux/1 -> Gain1/1
  variable lever term/1 -> Mux/2
  Sum1/1 -> Mux/1
  offset correction term/1 -> Sum1/1
  length change term/1 -> Sum1/2
  Constant2/1 -> Sum2/1
  Sum2/1 -> Gain5/1
  Constant1/1 -> Sum2/2, Sum3/1
  Sum3/1 -> Gain3/1
  phi23 [rad]/1 -> Sum3/2
  Product/1 -> Gain2/1
  Constant3/1 -> lever34 [m]/1, Product/2
  Sum4/1 -> Product/1
  Constant5/1 -> Sum4/2
  phi34 [rad]/1 -> Sum4/1
  Gain2/1 -> Sum5/1
  Gain4/1 -> Sum5/3
  Constant4/1 -> Sum5/2
  Sum5/1 -> lmtu [m]/1

== system nms_3Dmodel_inv_wAnkleCPG/NMC Model/Muscle Actuation Layer/L SOL ==
  note: Excitation Contraction Coupling
  note: SOL Muscle-Tendon Dynamics
  STIM : Inport
  lmtc [m] : Inport  Port=2
  1 : Product  Inputs=**  SaturateOnIntegerOverflow=on  InputSameDT=on  OutDataTypeStr=Inherit: Same as first input
  1/lslack : Gain  Gain=1/lslackSOL  SaturateOnIntegerOverflow=on  OutDataTypeStr=Inherit: Same as input  ParamDataTypeStr=Inherit: Same as input
  2 : Product  Inputs=***  SaturateOnIntegerOverflow=on  InputSameDT=on  OutDataTypeStr=Inherit: Same as first input
  BE force-length relation : Subsystem
  CE force-length relation : Subsystem
  CE inverse force-velocity relation : Subsystem
  Constant : Constant  Value=lslackSOL
  ECC TransferFcn : simulink_extras/Additional Linear/Transfer Fcn (with initial outputs)  N=[1]  D="[tau  1]"  Y0=preA  U0=0
      settings: AttributesFormatString=pre-activation: %<Y0>
  Fmax : Gain  Gain=FmaxSOL  SaturateOnIntegerOverflow=on  OutDataTypeStr=Inherit: Same as input  ParamDataTypeStr=Inherit: Same as input
  Fmax1 : Gain  Gain=FmaxSOL  SaturateOnIntegerOverflow=on  OutDataTypeStr=Inherit: Same as input  ParamDataTypeStr=Inherit: Same as input
  Fv = Fse / (A*Fce) : Product  Inputs=*/  SaturateOnIntegerOverflow=on  InputSameDT=on  OutDataTypeStr=Inherit: Same as first input
  Integrator : Integrator  InitialConditionSource=external  LowerSaturationLimit=0.05  ZeroCross=off
  PE force-length relation : Subsystem
  SE force-length relation : Subsystem
  Sum : Sum  Inputs=|+-  SaturateOnIntegerOverflow=on  InputSameDT=on  OutDataTypeStr=Inherit: Same as first input
  Sum2 : Sum  Inputs=|-+  SaturateOnIntegerOverflow=on  InputSameDT=on  OutDataTypeStr=Inherit: Same as first input
  Sum3 : Sum  SaturateOnIntegerOverflow=on  InputSameDT=on  OutDataTypeStr=Inherit: Same as first input
  Sum4 : Sum  SaturateOnIntegerOverflow=on  InputSameDT=on  OutDataTypeStr=Inherit: Same as first input
  lce/lopt : Gain  Gain=1/loptSOL  SaturateOnIntegerOverflow=on  OutDataTypeStr=Inherit: Same as input  ParamDataTypeStr=Inherit: Same as input
  vmax*lopt : Gain  Gain=vmaxSOL*loptSOL  SaturateOnIntegerOverflow=on  OutDataTypeStr=Inherit: Same as input  ParamDataTypeStr=Inherit: Same as input
  Fmtc : Outport  InitialOutput=0
  Lce : Outport  Port=2  InitialOutput=0
  Vce : Outport  Port=3  InitialOutput=0
  A : Outport  Port=4  InitialOutput=0
  Fac : Outport  Port=5  InitialOutput=0
  wires:
  Fmax1/1 -> Fac/1
  2/1 -> Fmax1/1
  ECC TransferFcn/1 -> 1/2, A/1, 2/2  "A"
  CE force-length relation/1(fce [Fmax]) -> 1/1, 2/1  "fl"
  Fv = Fse / (A*Fce)/1 -> CE inverse force-velocity relation/1(Fv[Fmax]), 2/3  "fv"
  STIM/1 -> ECC TransferFcn/1
  CE inverse force-velocity relation/1(v[vmax]) -> vmax*lopt/1
  Sum3/1 -> Fv = Fse / (A*Fce)/2
  BE force-length relation/1(fbe [Fmax]) -> Sum4/2
  1/1 -> Sum3/2
  PE force-length relation/1(fpe [Fmax]) -> Sum3/1
  Sum4/1 -> Fv = Fse / (A*Fce)/1
  Constant/1 -> Sum2/1
  Sum2/1 -> Integrator/2
  SE force-length relation/1(fse [Fmax]) -> Sum4/1, Fmax/1
  1/lslack/1 -> SE force-length relation/1(lse [lslack])
  Fmax/1 -> Fmtc/1  "Fmtc"
  lmtc [m]/1 -> Sum/1, Sum2/2  "lmtc"
  vmax*lopt/1 -> Vce/1, Integrator/1  "vce"
  lce/lopt/1 -> PE force-length relation/1(lce [lopt]), BE force-length relation/1(lce [lopt]), CE force-length relation/1(lce [lopt])
  Sum/1 -> 1/lslack/1  "lse"
  Integrator/1 -> Lce/1, lce/lopt/1, Sum/2  "lce"

== system nms_3Dmodel_inv_wAnkleCPG/NMC Model/Muscle Actuation Layer/L SOL Link ==
  note: Soleus Attachment
  phi12 [rad] : Inport
  Constant : Constant  Value=lslackSOL+loptSOL
  Constant3 : Constant  Value=phimaxSOL
  Constant5 : Constant  Value=phirefSOL
  Demux1 : Demux  Outputs=2
  Gain2 : Gain  Gain=rSOLmax
  Gain3 : Gain  Gain=phiScaleSOL
  Gain8 : Gain  Gain=phiScaleSOL
  Gain9 : Gain  Gain=rhoSOL/phiScaleSOL
  Mux1 : Mux  Inputs=2
  Sum4 : Sum  Inputs=-+
  Sum5 : Sum  Inputs=|+-
  Sum6 : Sum  Inputs=|+-
  Sum7 : Sum  Inputs=-+|
  length change term1 : Trigonometry
  offset correction term1 : Trigonometry
  variable lever term1 : Trigonometry  Operator=cos
  lmtc [m] : Outport
  lever [m] : Outport  Port=2
  wires:
  Gain8/1 -> offset correction term1/1
  Gain3/1 -> length change term1/1, variable lever term1/1
  Gain2/1 -> Demux1/1
  Mux1/1 -> Gain2/1
  variable lever term1/1 -> Mux1/2
  Sum4/1 -> Mux1/1
  offset correction term1/1 -> Sum4/1
  length change term1/1 -> Sum4/2
  Constant5/1 -> Sum6/1
  Sum6/1 -> Gain8/1
  Constant3/1 -> Sum6/2, Sum7/1
  Sum7/1 -> Gain3/1
  phi12 [rad]/1 -> Sum7/2
  Demux1/2 -> lever [m]/1
  Demux1/1 -> Gain9/1
  Gain9/1 -> Sum5/2
  Sum5/1 -> lmtc [m]/1
  Constant/1 -> Sum5/1

== system nms_3Dmodel_inv_wAnkleCPG/NMC Model/Muscle Actuation Layer/L TA ==
  note: TA Muscle-Tendon Dynamics
  note: Excitation Contraction Coupling
  STIM : Inport
  lmtc [m] : Inport  Port=2
  1 : Product  Inputs=**  SaturateOnIntegerOverflow=on  InputSameDT=on  OutDataTypeStr=Inherit: Same as first input
  1/lslack : Gain  Gain=1/lslackTA  SaturateOnIntegerOverflow=on  OutDataTypeStr=Inherit: Same as input  ParamDataTypeStr=Inherit: Same as input
  2 : Product  Inputs=***  SaturateOnIntegerOverflow=on  InputSameDT=on  OutDataTypeStr=Inherit: Same as first input
  BE force-length relation : Subsystem
  CE force-length relation : Subsystem
  CE inverse force-velocity relation : Subsystem
  Constant : Constant  Value=lslackTA
  ECC TransferFcn : simulink_extras/Additional Linear/Transfer Fcn (with initial outputs)  N=[1]  D="[tau  1]"  Y0=preA  U0=0
      settings: AttributesFormatString=pre-activation: %<Y0>
  Fmax : Gain  Gain=FmaxTA  SaturateOnIntegerOverflow=on  OutDataTypeStr=Inherit: Same as input  ParamDataTypeStr=Inherit: Same as input
  Fmax1 : Gain  Gain=FmaxTA  SaturateOnIntegerOverflow=on  OutDataTypeStr=Inherit: Same as input  ParamDataTypeStr=Inherit: Same as input
  Fv = Fse / (A*Fce) : Product  Inputs=*/  SaturateOnIntegerOverflow=on  InputSameDT=on  OutDataTypeStr=Inherit: Same as first input
  Integrator : Integrator  InitialConditionSource=external  LowerSaturationLimit=0.05  ZeroCross=off
  PE force-length relation : Subsystem
  SE force-length relation : Subsystem
  Sum : Sum  Inputs=|+-  SaturateOnIntegerOverflow=on  InputSameDT=on  OutDataTypeStr=Inherit: Same as first input
  Sum2 : Sum  Inputs=|-+  SaturateOnIntegerOverflow=on  InputSameDT=on  OutDataTypeStr=Inherit: Same as first input
  Sum3 : Sum  SaturateOnIntegerOverflow=on  InputSameDT=on  OutDataTypeStr=Inherit: Same as first input
  Sum4 : Sum  SaturateOnIntegerOverflow=on  InputSameDT=on  OutDataTypeStr=Inherit: Same as first input
  lce/lopt : Gain  Gain=1/loptTA  SaturateOnIntegerOverflow=on  OutDataTypeStr=Inherit: Same as input  ParamDataTypeStr=Inherit: Same as input
  vmax*lopt : Gain  Gain=vmaxTA*loptTA  SaturateOnIntegerOverflow=on  OutDataTypeStr=Inherit: Same as input  ParamDataTypeStr=Inherit: Same as input
  Fmtc : Outport  InitialOutput=0
  Lce : Outport  Port=2  InitialOutput=0
  Vce : Outport  Port=3  InitialOutput=0
  A : Outport  Port=4  InitialOutput=0
  Fac : Outport  Port=5  InitialOutput=0
  wires:
  Fmax1/1 -> Fac/1
  2/1 -> Fmax1/1
  ECC TransferFcn/1 -> A/1, 2/2, 1/2  "A"
  Fv = Fse / (A*Fce)/1 -> CE inverse force-velocity relation/1(Fv[Fmax]), 2/3  "fv"
  STIM/1 -> ECC TransferFcn/1
  Integrator/1 -> Lce/1, Sum/2, lce/lopt/1  "lce"
  Sum/1 -> 1/lslack/1  "lse"
  lce/lopt/1 -> CE force-length relation/1(lce [lopt]), PE force-length relation/1(lce [lopt]), BE force-length relation/1(lce [lopt])
  vmax*lopt/1 -> Vce/1, Integrator/1  "vce"
  lmtc [m]/1 -> Sum2/2, Sum/1  "lmtc"
  Fmax/1 -> Fmtc/1  "Fmtc"
  1/lslack/1 -> SE force-length relation/1(lse [lslack])
  SE force-length relation/1(fse [Fmax]) -> Fmax/1, Sum4/1
  Sum2/1 -> Integrator/2
  Constant/1 -> Sum2/1
  CE force-length relation/1(fce [Fmax]) -> 1/1, 2/1
  Sum4/1 -> Fv = Fse / (A*Fce)/1
  PE force-length relation/1(fpe [Fmax]) -> Sum3/1
  1/1 -> Sum3/2
  BE force-length relation/1(fbe [Fmax]) -> Sum4/2
  Sum3/1 -> Fv = Fse / (A*Fce)/2
  CE inverse force-velocity relation/1(v[vmax]) -> vmax*lopt/1

== system nms_3Dmodel_inv_wAnkleCPG/NMC Model/Muscle Actuation Layer/L TA Link ==
  note: Muscle Length and Moment Arm
  phi12 [rad] : Inport
  Constant : Constant  Value=lslackTA+loptTA
  Constant3 : Constant  Value=phimaxTA
  Constant5 : Constant  Value=phirefTA
  Demux1 : Demux  Outputs=2
  Gain2 : Gain  Gain=rTAmax
  Gain3 : Gain  Gain=phiScaleTA
  Gain8 : Gain  Gain=phiScaleTA
  Gain9 : Gain  Gain=rhoTA/phiScaleTA
  Mux1 : Mux  Inputs=2
  Sum4 : Sum  Inputs=-+
  Sum5 : Sum  Inputs=|++
  Sum6 : Sum  Inputs=|+-
  Sum7 : Sum  Inputs=-+|
  length change term1 : Trigonometry
  offset correction term1 : Trigonometry
  variable lever term1 : Trigonometry  Operator=cos
  lmtc [m] : Outport
  lever [m] : Outport  Port=2
  wires:
  Gain8/1 -> offset correction term1/1
  Gain3/1 -> length change term1/1, variable lever term1/1
  Gain2/1 -> Demux1/1
  Mux1/1 -> Gain2/1
  variable lever term1/1 -> Mux1/2
  Sum4/1 -> Mux1/1
  offset correction term1/1 -> Sum4/1
  length change term1/1 -> Sum4/2
  Constant5/1 -> Sum6/1
  Sum6/1 -> Gain8/1
  Constant3/1 -> Sum6/2, Sum7/1
  Sum7/1 -> Gain3/1
  phi12 [rad]/1 -> Sum7/2
  Demux1/2 -> lever [m]/1
  Demux1/1 -> Gain9/1
  Gain9/1 -> Sum5/2
  Sum5/1 -> lmtc [m]/1
  Constant/1 -> Sum5/1

== system nms_3Dmodel_inv_wAnkleCPG/NMC Model/Muscle Actuation Layer/L VAS ==
  note: Excitation Contraction Coupling
  note: VAS Muscle-Tendon Dynamics
  STIM : Inport
  lmtc [m] : Inport  Port=2
  1 : Product  Inputs=**  SaturateOnIntegerOverflow=on  InputSameDT=on  OutDataTypeStr=Inherit: Same as first input
  1/lslack : Gain  Gain=1/lslackVAS  SaturateOnIntegerOverflow=on  OutDataTypeStr=Inherit: Same as input  ParamDataTypeStr=Inherit: Same as input
  2 : Product  Inputs=***  SaturateOnIntegerOverflow=on  InputSameDT=on  OutDataTypeStr=Inherit: Same as first input
  BE force-length relation : Subsystem
  CE force-length relation : Subsystem
  CE inverse force-velocity relation : Subsystem
  Constant : Constant  Value=lslackVAS
  ECC TransferFcn : simulink_extras/Additional Linear/Transfer Fcn (with initial outputs)  N=[1]  D="[tau  1]"  Y0=preA  U0=0
      settings: AttributesFormatString=pre-activation: %<Y0>
  Fmax : Gain  Gain=FmaxVAS  SaturateOnIntegerOverflow=on  OutDataTypeStr=Inherit: Same as input  ParamDataTypeStr=Inherit: Same as input
  Fmax1 : Gain  Gain=FmaxVAS  SaturateOnIntegerOverflow=on  OutDataTypeStr=Inherit: Same as input  ParamDataTypeStr=Inherit: Same as input
  Fv = Fse / (A*Fce) : Product  Inputs=*/  SaturateOnIntegerOverflow=on  InputSameDT=on  OutDataTypeStr=Inherit: Same as first input
  Integrator : Integrator  InitialConditionSource=external  LowerSaturationLimit=0.05  ZeroCross=off
  PE force-length relation : Subsystem
  SE force-length relation : Subsystem
  Sum : Sum  Inputs=|+-  SaturateOnIntegerOverflow=on  InputSameDT=on  OutDataTypeStr=Inherit: Same as first input
  Sum2 : Sum  Inputs=|-+  SaturateOnIntegerOverflow=on  InputSameDT=on  OutDataTypeStr=Inherit: Same as first input
  Sum3 : Sum  SaturateOnIntegerOverflow=on  InputSameDT=on  OutDataTypeStr=Inherit: Same as first input
  Sum4 : Sum  SaturateOnIntegerOverflow=on  InputSameDT=on  OutDataTypeStr=Inherit: Same as first input
  lce/lopt : Gain  Gain=1/loptVAS  SaturateOnIntegerOverflow=on  OutDataTypeStr=Inherit: Same as input  ParamDataTypeStr=Inherit: Same as input
  vmax*lopt : Gain  Gain=vmaxVAS*loptVAS  SaturateOnIntegerOverflow=on  OutDataTypeStr=Inherit: Same as input  ParamDataTypeStr=Inherit: Same as input
  Fmtc : Outport  InitialOutput=0
  Lce : Outport  Port=2  InitialOutput=0
  Vce : Outport  Port=3  InitialOutput=0
  A : Outport  Port=4  InitialOutput=0
  Fac : Outport  Port=5  InitialOutput=0
  wires:
  Fmax1/1 -> Fac/1
  2/1 -> Fmax1/1
  ECC TransferFcn/1 -> A/1, 2/2, 1/2  "fl"
  Fv = Fse / (A*Fce)/1 -> CE inverse force-velocity relation/1(Fv[Fmax]), 2/3  "fv"
  STIM/1 -> ECC TransferFcn/1
  CE inverse force-velocity relation/1(v[vmax]) -> vmax*lopt/1
  Sum3/1 -> Fv = Fse / (A*Fce)/2
  BE force-length relation/1(fbe [Fmax]) -> Sum4/2
  1/1 -> Sum3/2
  PE force-length relation/1(fpe [Fmax]) -> Sum3/1
  Sum4/1 -> Fv = Fse / (A*Fce)/1
  CE force-length relation/1(fce [Fmax]) -> 1/1, 2/1
  Constant/1 -> Sum2/1
  Sum2/1 -> Integrator/2
  SE force-length relation/1(fse [Fmax]) -> Sum4/1, Fmax/1
  1/lslack/1 -> SE force-length relation/1(lse [lslack])
  Fmax/1 -> Fmtc/1  "Fmtc"
  lmtc [m]/1 -> Sum/1, Sum2/2  "lmtc"
  vmax*lopt/1 -> Vce/1, Integrator/1  "vce"
  lce/lopt/1 -> PE force-length relation/1(lce [lopt]), BE force-length relation/1(lce [lopt]), CE force-length relation/1(lce [lopt])
  Sum/1 -> 1/lslack/1  "lse"
  Integrator/1 -> Lce/1, lce/lopt/1, Sum/2  "lce"

== system nms_3Dmodel_inv_wAnkleCPG/NMC Model/Muscle Actuation Layer/L VAS Link ==
  note: Muscle Length and Moment Arm
  phi23 [rad] : Inport
  Constant : Constant  Value=lslackVAS+loptVAS
  Constant1 : Constant  Value=phimaxVAS
  Constant2 : Constant  Value=phirefVAS
  Demux : Demux  Outputs=2
  Gain1 : Gain  Gain=rVASmax
  Gain3 : Gain  Gain=phiScaleVAS
  Gain4 : Gain  Gain=rhoVAS/phiScaleVAS
  Gain5 : Gain  Gain=phiScaleVAS
  Mux : Mux  Inputs=2
  Sum1 : Sum  Inputs=-+
  Sum2 : Sum  Inputs=|+-
  Sum3 : Sum  Inputs=-+|
  Sum5 : Sum  Inputs=|+-
  length change term : Trigonometry
  offset correction term : Trigonometry
  variable lever term : Trigonometry  Operator=cos
  lmtu [m] : Outport
  lever [m] : Outport  Port=2
  wires:
  Gain4/1 -> Sum5/2
  Gain5/1 -> offset correction term/1
  Gain3/1 -> length change term/1, variable lever term/1
  Demux/1 -> Gain4/1
  Demux/2 -> lever [m]/1
  Gain1/1 -> Demux/1
  Mux/1 -> Gain1/1
  variable lever term/1 -> Mux/2
  Sum1/1 -> Mux/1
  offset correction term/1 -> Sum1/1
  length change term/1 -> Sum1/2
  Constant2/1 -> Sum2/1
  Sum2/1 -> Gain5/1
  Constant1/1 -> Sum2/2, Sum3/1
  Sum3/1 -> Gain3/1
  phi23 [rad]/1 -> Sum3/2
  Sum5/1 -> lmtu [m]/1
  Constant/1 -> Sum5/1

== system nms_3Dmodel_inv_wAnkleCPG/NMC Model/Muscle Actuation Layer/Metabolic Energy LBFSH ==
  Constant : Constant  Value=loptBFSH
  Constant1 : Constant  Value=massBFSH
  Constant2 : Constant  Value=t1fBFSH
  Metabolic Energy : nmc/Metabolic Energy
  tag scope: LEnergyBFSH=global
  wires:
  [LActBFSH] -> Metabolic Energy/1
  [LStimBFSH] -> Metabolic Energy/2
  [LLceBFSH] -> Metabolic Energy/3
  [LVceBFSH] -> Metabolic Energy/4
  [LFmBFSH] -> Metabolic Energy/5
  [LFactBFSH] -> Metabolic Energy/6
  Constant/1 -> Metabolic Energy/7
  Constant1/1 -> Metabolic Energy/8
  Constant2/1 -> Metabolic Energy/9
  Metabolic Energy/1 -> [LEnergyBFSH]
